simulink library "Vex-V5-Simulink-Expansion"  (R2022a)
settings: Solver=VariableStepAuto  StartTime=0.0  StopTime=10.0  RelTol=1e-3
libraries: $bdroot x48, vexv5lib x31, dspsigops x6, dsparch4 x2, slpidlib x1
(part 1 of 2)
settings Model: Creator=ronan  LastModifiedBy=ronan

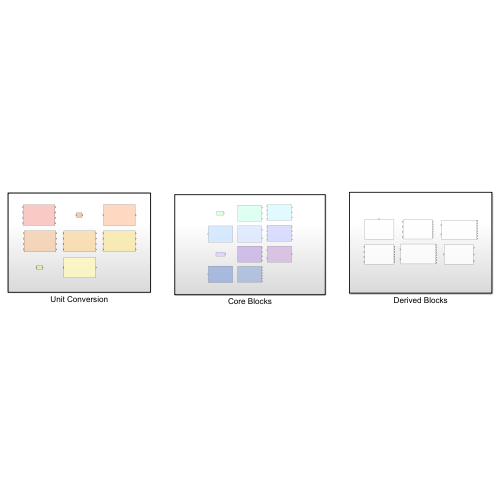
[thumbnail: Simulink's stored preview of the top-level diagram]
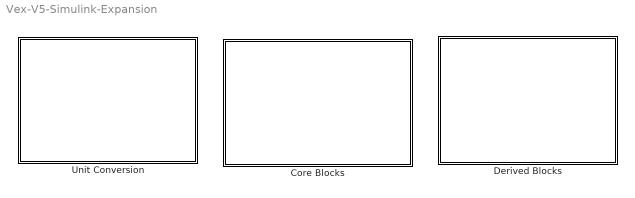
== system Vex-V5-Simulink-Expansion ==
  Core Blocks : Subsystem
  Derived Blocks : Subsystem
  Unit Conversion : Subsystem

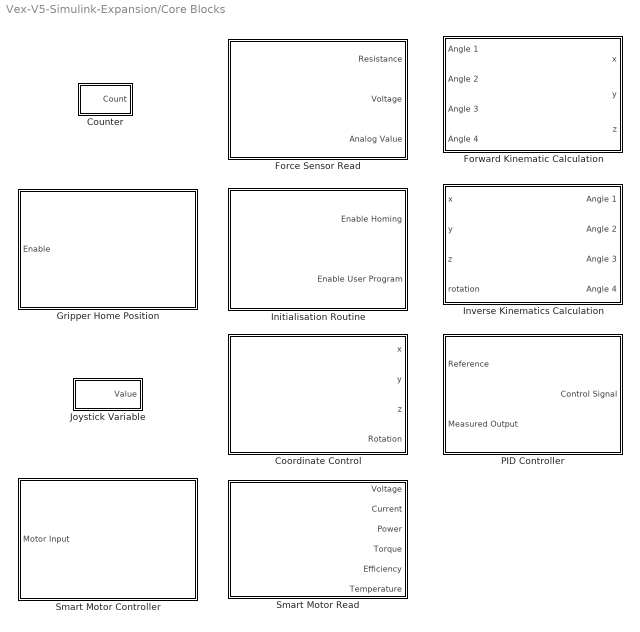
== system Vex-V5-Simulink-Expansion/Core Blocks ==
  Coordinate Control : Subsystem  mask(Coordinate Control){SampleTime=0.01, GX=0, GY=0, GZ=0, GR=0, IX=150, IY=0, IZ=120, IR=85}
      mask prompts: SampleTime "Sample time:"; GX "x (mm/s):"; GY "y (mm/s):"; GZ "z (mm/s):"; GR "Rotation (deg/s):"; IX "x (mm):"; IY "y (mm):"; IZ "z (mm):"; IR "Rotation (deg):"
      mask help: Allows the use of the Vex Joystick's analog sticks as a means to control a Cartesian coordinate and a rotation. This is typically used with the 'Inverse Kinematics Motion' block to allow for manual movement.
      mask TypeOptions SampleTime: Gamepad Joystick/SampleTime | Gamepad Joystick1/SampleTime | Gamepad Joystick2/SampleTime | Gamepad Joystick3/SampleTime
      mask DialogControl ParameterGroupVar Prompt: Global Parameters
      mask DialogControl Container3 Prompt: Maximum Movement Rate
      mask DialogControl Container4 Prompt: Initial Conditions
      mask Display:
      | disp('Coordinate Control');
      | port_label('output', 1, 'x');
      | port_label('output', 2, 'y');
      | port_label('output', 3, 'z');
      | port_label('output', 4, 'Rotation');
  Counter : Subsystem  mask(Counter){SampleTime=0.01, cycleTime=5, cycles=2}
      mask prompts: SampleTime "Sample Time:"; cycleTime "Cycle Time (s):"; cycles "Number of Cycles:"
      mask help: Counts from 1 to the specified limit with the given cycle time before resetting. Outputs the current count.
      mask TypeOptions SampleTime: Delay/SampleTime | Delay1/SampleTime
      mask Display: disp(['Counter']);
  Force Sensor Read : Subsystem  mask(Force Sensor Read){port=H, SampleTime=0.01, Value=22000}
      mask prompts: SampleTime "Sample time:"; Value "Resistance:"
      mask help: Reads the analog input corresponding to the force sensor, and returns the input voltage and the sensor's resistance.
      mask TypeOptions port: Force Sensor Input/port
      mask TypeOptions SampleTime: Force Sensor Input/SampleTime
      mask TypeOptions Value: Resistor Value/Value
      mask DialogControl ParameterGroupVar Prompt: Force Sensor Input
      mask DialogControl Container3 Prompt: Circuit Parameters
      mask Display:
      | port = get_param(gcb, 'port');
      | text(0.4,0.45, ['Input ',port]);
      | text(0.25,0.55, 'Force Sensor Read');
      | port_label('output', 1, 'Resistance');
      | port_label('output', 2, 'Voltage');
      | port_label('output', 3, 'Analog Value');
  Forward Kinematic Calculation : Subsystem  mask(Forward Kinematic Calculation){}
      mask help: Calculates the Cartesian coordinate (mm) of the end effector for a set of motor angles (radians).
      mask Display:
      | disp('Forward Kinematic Calculation');
      | 
      | port_label('output', 1, 'x');
      | port_label('output', 2, 'y');
      | port_label('output', 3, 'z');
      | 
      | port_label('input', 1, 'Angle A');
      | port_label('input', 2, 'Angle B');
      | port_label('input', 3, 'Angle C');
      | port_label('input', 4, 'Angle D');
  Gripper Home Position : Subsystem  mask(Gripper Home Position){SampleTime=0.01, motorPort_right=6, motorPort_left=5}
      mask prompts: SampleTime "Sample Time:"; motorPort_right "Right Gripper:"; motorPort_left "Left Gripper:"
      mask help: Given an enable input, moves the gripper to the home position and resets the motor encoders.
      mask TypeOptions motorPort_right: Subsystem/Right Gripper Read/motorPort | Subsystem/Right Gripper Write/motorPort
      mask TypeOptions motorPort_left: Subsystem/Left Gripper Read/motorPort | Subsystem/Left Gripper Write/motorPort
      mask DialogControl ParameterGroupVar Prompt: Global Parameters
      mask DialogControl Container3 Prompt: Smart Motor Ports
  Initialisation Routine : Subsystem  mask(Initialisation Routine){}
      mask help: Used to home the Vex Arm prior to beginning the User Program - default setting is 5 seconds.
  Inverse Kinematics Calculation : Subsystem  mask(Inverse Kinematics){}
      mask help: Calculates the required motor angles to reach the input end effector rotation (radians) and Cartesian coordinate (mm).
      mask Display:
      | disp('Inverse Kinematic Calculation');
      | 
      | port_label('output', 1, 'Angle A');
      | port_label('output', 2, 'Angle B');
      | port_label('output', 3, 'Angle C');
      | port_label('output', 4, 'Angle D');
      | 
      | port_label('input', 1, 'x');
      | port_label('input', 2, 'y');
      | port_label('input', 3, 'z');
      | port_label('input', 4, 'Rotation');
  Joystick Variable : Subsystem  mask(Joystick Variable){chan_inc=R1, chan_dec=R2, SampleTime=0.01, rate=0, init=0, max=1, min=-1}
      mask prompts: chan_inc "Increment Button:"; chan_dec "Decrement Button:"; SampleTime "Sample time:"; rate "Rate (1/s):"; init "Initial Value:"; max "Maximum Value:"; min "Minimum Value:"
      mask help: Allows a variable to be incremented/decremented using two specified buttons on the Vex Joystick. The rate of change and limits can also be selected.
      mask TypeOptions chan_inc: Gamepad Button Increment/chan
      mask TypeOptions chan_dec: Gamepad Button Decrement/chan
      mask TypeOptions SampleTime: Gamepad Button Decrement/SampleTime | Gamepad Button Increment/SampleTime
      mask DialogControl ParameterGroupVar Prompt: Joystick Parameters
      mask DialogControl Container3 Prompt: Variable Parameters
      mask Display: disp('Variable');
  PID Controller : Subsystem  mask(PID Controller){KP=0, KI=0, KD=0, LimitOutput=off, limitHigh=0, limitLow=0, AntiWindupMode=none, kb=0}
      mask prompts: KP "Proportional (P):"; KI "Integral (I):"; KD "Derivative (D):"; LimitOutput "Simulink:masks:LimitOutput_MP"; limitHigh "Upper limit:"; limitLow "Lower limit:"; AntiWindupMode "Simulink:masks:AntiwindupMethod_MP"; kb "Back-calculation coefficient (Kb):"
      mask help: A general PID controller requiring an input reference and measured value.
      mask TypeOptions LimitOutput: PID/LimitOutput
      mask Callback limitHigh:
      | % Get path to PID controller block
      |     path = strcat(gcb, '/PID');
      |     % Load mask and PID parameters
      |     limMask = get_param(gcb, 'limitHigh');
      |     t = Simulink.Mask.get(path);
      |     limH = t.getParameter('UpperSaturationLimit');
      |     % Set PID limit to mask value
      |     limH.Value = limMask;
      mask Callback limitLow:
      | % Get path to PID controller block
      |     path = strcat(gcb, '/PID');
      |     % Load mask and PID parameters
      |     limMask = get_param(gcb, 'limitLow');
      |     t = Simulink.Mask.get(path);
      |     limL = t.getParameter('LowerSaturationLimit');
      |     % Set PID limit to mask value
      |     limL.Value = limMask;
      mask TypeOptions AntiWindupMode: PID/AntiWindupMode
      mask Callback AntiWindupMode:
      | %{
      |     limMask = get_param(gcb, 'limitOutput');
      |     m = Simulink.Mask.get(gcb);
      |     antiwind = m.getParameter('AntiWindupMode');
      |     kb = m.getParameter('kb');
      |     if strcmp(antiwind.Value,'back-calculation')
      |         if strcmp(limMask,'on')
      |             kb.Enabled = 'on';
      |         end
      |     else
      |         kb.Enabled = 'off';
      |     end
      | %}
      mask Callback kb:
      | % Get path to PID controller block
      |     path = strcat(gcb, '/PID');
      |     % Load mask and PID parameters
      |     kbMask = get_param(gcb, 'kb');
      |     t = Simulink.Mask.get(path);
      |     kbPID = t.getParameter('Kb');
      |     kbPID.Value = kbMask;
      mask DialogControl Container3 Prompt: Controller Parameters
      mask DialogControl ParameterGroupVar Prompt: Output Saturation
      mask DialogControl LimitOutput Prompt: Limit output
      mask DialogControl AntiWindupMode Prompt: Anti-windup Method:
      mask Display:
      | port_label('output', 1, 'Control Signal');
      | port_label('input', 1, 'Reference');
      | port_label('input', 2, 'Measured Output');
      | 
      | kp = get_param(gcb, 'KP');
      | text(0.15,0.1,['KP: ',kp])
      | 
      | ki = get_param(gcb, 'KI');
      | text(0.45,0.1,['KI: ',ki])
      | 
      | kd = get_param(gcb, 'KD');
      | text(0.75,0.1,['KD: ',kd])
  Smart Motor Controller : Subsystem  mask(Smart Motor Controller){motorPort=1, OperationMode=Advanced Control, MotorBrakeMode=Coast}
      mask prompts: motorPort "Smart Port:"; OperationMode "Control Mode:"; MotorBrakeMode "Braking Mode:"
      mask help: Controls the Vex Smart Motor via the chosen method.
      mask TypeOptions motorPort: MATLAB System/motorPort
      mask TypeOptions OperationMode: MATLAB System/OperationMode
      mask TypeOptions MotorBrakeMode: MATLAB System/MotorBrakeMode
      mask DialogControl Container3 Prompt: Smart Motor Configuration
      mask Display:
      | %mode = get_param(gcb, 'control');
      | port = get_param(gcb, 'motorPort');
      | %text(0.3,0.45,[mode]);
      | 
      | text(0.5,0.5, 'Smart Motor Controller','HorizontalAlignment','center');
      | text(0.42,0.15, ['Port: ',port]);
  Smart Motor Read : Subsystem  mask(Smart Motor Read){motorPort=1, SampleTime=0.01}
      mask prompts: motorPort "Smart Port:"; SampleTime "Sample time:"
      mask help: This block reads several attributes relating to the Vex Smart Motors for use in control.
      mask TypeOptions motorPort: MATLAB System1/motorPort
      mask TypeOptions SampleTime: MATLAB System1/SampleTime
      mask Display:
      | port_label('output', 1, 'Voltage');
      | port_label('output', 2, 'Current');
      | port_label('output', 3, 'Power');
      | port_label('output', 4, 'Torque');
      | port_label('output', 5, 'Efficiency');
      | port_label('output', 6, 'Temperature');
      | 
      | text(0.5,0.5,'Smart Motor Read','HorizontalAlignment','center')
      | port = get_param(gcb, 'motorPort');
      | text(0.42,0.15, ['Port: ',port]);

== system Vex-V5-Simulink-Expansion/Derived Blocks ==
  Arm Home Position : Subsystem  mask(Home Position){home_A=0, home_B=0, home_C=0, home_D=0, SampleTime=0.01}
      mask prompts: home_A "Joint A:"; home_B "Joint B:"; home_C "Joint C:"; home_D "Joint D:"; SampleTime "Sample Time:"
      mask help: Moves the Vex Arm into the specified home position prior to executing the user program.
      mask DialogControl ParameterGroupVar Prompt: Potentiometer Home Readings
      mask DialogControl Container3 Prompt: Global Parameters
  Forward Kinematic Motion : Subsystem  mask(Forward Kinematic Motion){SampleTime=0.01, OperationMode=Advanced Control, MotorBrakeMode=Coast, Home_A=0, Home_B=0, Home_C=0, Home_D=0, KP_A=0, KI_A=0, KD_A=0, LimitOutput_A=off, limitHigh_A=0, limitLow_A=0, AntiWindupMode_A=none, kb_A=0, KP_B=0, KI_B=0, KD_B=0, LimitOutput_B=off, limitHigh_B=0, limitLow_B=0, AntiWindupMode_B=none, kb_B=0, KP_C=0, KI_C=0, KD_C=0, LimitOutput_C=off, limitHigh_C=0, limitLow_C=0, AntiWindupMode_C=none, kb_C=0, KP_D=0, KI_D=0, KD_D=0, LimitOutput_D=off, limitHigh_D=0, limitLow_D=0, AntiWindupMode_D=none, kb_D=0}
      mask prompts: SampleTime "Sample Time:"; OperationMode "Control Mode:"; MotorBrakeMode "Braking Mode:"; Home_A "Joint A:"; Home_B "Joint B:"; Home_C "Joint C:"; Home_D "Joint D:"; KP_A "Proportional (P):"; KI_A "Integral (I):"; KD_A "Derivative (D):"; LimitOutput_A "Simulink:masks:LimitOutput_MP"; limitHigh_A "Upper limit:"; limitLow_A "Lower limit:"; AntiWindupMode_A "Simulink:masks:AntiwindupMethod_MP"; kb_A "Back-calculation coefficient (Kb):"; KP_B "Proportional (P):"; KI_B "Integral (I):"; KD_B "Derivative (D):"; LimitOutput_B "Simulink:masks:LimitOutput_MP"; limitHigh_B "Upper limit:"; limitLow_B "Lower limit:"; AntiWindupMode_B "Simulink:masks:AntiwindupMethod_MP"; kb_B "Back-calculation coefficient (Kb):"; KP_C "Proportional (P):"; KI_C "Integral (I):"; KD_C "Derivative (D):"; LimitOutput_C "Simulink:masks:LimitOutput_MP"; limitHigh_C "Upper limit:"; limitLow_C "Lower limit:"; AntiWindupMode_C "Simulink:masks:AntiwindupMethod_MP"; kb_C "Back-calculation coefficient (Kb):"; KP_D "Proportional (P):"; KI_D "Integral (I):"; KD_D "Derivative (D):"; LimitOutput_D "Simulink:masks:LimitOutput_MP"; limitHigh_D "Upper limit:"; limitLow_D "Lower limit:"; AntiWindupMode_D "Simulink:masks:AntiwindupMethod_MP"; kb_D "Back-calculation coefficient (Kb):"
      mask help: Given a set of 4 arm angles (radians), moves the arm into that position using the selected PID control parameters and outputs the current pose and Cartesian coordinate of the end effector (mm).
      mask TypeOptions OperationMode: Smart Motor Controller A/OperationMode | Smart Motor Controller B/OperationMode | Smart Motor Controller C/OperationMode | Smart Motor Controller D/OperationMode
      mask TypeOptions MotorBrakeMode: Smart Motor Controller A/MotorBrakeMode | Smart Motor Controller B/MotorBrakeMode | Smart Motor Controller C/MotorBrakeMode | Smart Motor Controller D/MotorBrakeMode
      mask TypeOptions Home_A: A2P/Home_A | P2A/Home_A
      mask TypeOptions Home_B: A2P/Home_B | P2A/Home_B
      mask TypeOptions Home_C: A2P/Home_C | P2A/Home_C
      mask TypeOptions Home_D: A2P/Home_D | P2A/Home_D
      mask TypeOptions KP_A: PID Controller A/KP
      mask TypeOptions KI_A: PID Controller A/KI
      mask TypeOptions KD_A: PID Controller A/KD
      mask TypeOptions LimitOutput_A: PID Controller A/LimitOutput
      mask TypeOptions limitHigh_A: PID Controller A/limitHigh
      mask TypeOptions limitLow_A: PID Controller A/limitLow
      mask TypeOptions AntiWindupMode_A: PID Controller A/AntiWindupMode
      mask TypeOptions kb_A: PID Controller A/kb
      mask TypeOptions KP_B: PID Controller B/KP
      mask TypeOptions KI_B: PID Controller B/KI
      mask TypeOptions KD_B: PID Controller B/KD
      mask TypeOptions LimitOutput_B: PID Controller B/LimitOutput
      mask TypeOptions limitHigh_B: PID Controller B/limitHigh
      mask TypeOptions limitLow_B: PID Controller B/limitLow
      mask TypeOptions AntiWindupMode_B: PID Controller B/AntiWindupMode
      mask TypeOptions kb_B: PID Controller B/kb
      mask TypeOptions KP_C: PID Controller C/KP
      mask TypeOptions KI_C: PID Controller C/KI
      mask TypeOptions KD_C: PID Controller C/KD
      mask TypeOptions LimitOutput_C: PID Controller C/LimitOutput
      mask TypeOptions limitHigh_C: PID Controller C/limitHigh
      mask TypeOptions limitLow_C: PID Controller C/limitLow
      mask TypeOptions AntiWindupMode_C: PID Controller C/AntiWindupMode
      mask TypeOptions kb_C: PID Controller C/kb
      mask TypeOptions KP_D: PID Controller D/KP
      mask TypeOptions KI_D: PID Controller D/KI
      mask TypeOptions KD_D: PID Controller D/KD
      mask TypeOptions LimitOutput_D: PID Controller D/LimitOutput
      mask TypeOptions limitHigh_D: PID Controller D/limitHigh
      mask TypeOptions limitLow_D: PID Controller D/limitLow
      mask TypeOptions AntiWindupMode_D: PID Controller D/AntiWindupMode
      mask TypeOptions kb_D: PID Controller D/kb
      mask DialogControl Container17 Prompt: Global Parameters
      mask DialogControl Container16 Prompt: Global Motor Parameters
      mask DialogControl Container15 Prompt: Potentiometer Home Values
      mask DialogControl Container3 Prompt: PID Controller A
      mask DialogControl Container7 Prompt: PID Gains
      mask DialogControl Container8 Prompt: Output Saturation
      mask DialogControl LimitOutput_A Prompt: Limit output
      mask DialogControl AntiWindupMode_A Prompt: Anti-windup Method:
      mask DialogControl Container4 Prompt: PID Controller B
      mask DialogControl Container9 Prompt: PID Gains
      mask DialogControl Container10 Prompt: Output Saturation
      mask DialogControl LimitOutput_B Prompt: Limit output
      mask DialogControl AntiWindupMode_B Prompt: Anti-windup Method:
      mask DialogControl Container5 Prompt: PID Controller C
      mask DialogControl Container11 Prompt: PID Gains
      mask DialogControl Container12 Prompt: Output Saturation
      mask DialogControl LimitOutput_C Prompt: Limit output
      mask DialogControl AntiWindupMode_C Prompt: Anti-windup Method:
      mask DialogControl Container6 Prompt: PID Controller D
      mask DialogControl Container13 Prompt: PID Gains
      mask DialogControl Container14 Prompt: Output Saturation
      mask DialogControl LimitOutput_D Prompt: Limit output
      mask DialogControl AntiWindupMode_D Prompt: Anti-windup Method:
  Individual Gripper Control : Subsystem  mask(Individual Gripper Control){SampleTime=0.01, motorPort_right=5, motorPort_left=6, KP=0, KI=0, KD=0, LimitOutput=off, limitHigh=0, limitLow=0, AntiWindupMode=none, kb=0, fsr_unit=Resistance, port_LA=A, LA=47000, port_LB=B, LB=47000, port_RA=D, RA=47000, port_RB=C, RB=47000}
      mask prompts: SampleTime "Sample Time:"; motorPort_right "Right Smart Port:"; motorPort_left "Left Smart Port:"; KP "Proportional (P):"; KI "Integral (I):"; KD "Derivative (D):"; LimitOutput "Simulink:masks:LimitOutput_MP"; limitHigh "Upper limit:"; limitLow "Lower limit:"; AntiWindupMode "Simulink:masks:AntiwindupMethod_MP"; kb "Back-calculation coefficient (Kb):"; fsr_unit "Output Unit:"; port_LA "Port:"; LA "Resistance:"; port_LB "Port:"; LB "Resistance:"; port_RA "Port:"; RA "Resistance:"; port_RB "Port:"; RB "Resistance:"
      mask help: Allows control of each gripper arm's position via a reference angle and PID parameters. Returns force sensor readings, the current motor encoder positions and the measured torque.
      mask TypeOptions motorPort_right: Right Smart Motor Controller/motorPort | Smart Motor Read Right/motorPort
      mask TypeOptions motorPort_left: Left Smart Motor Controller/motorPort | Smart Motor Read Left/motorPort
      mask TypeOptions KP: PID Controller Left/KP | PID Controller Right/KP
      mask TypeOptions KI: PID Controller Left/KI | PID Controller Right/KI
      mask TypeOptions KD: PID Controller Left/KD | PID Controller Right/KD
      mask TypeOptions LimitOutput: PID Controller Left/LimitOutput | PID Controller Right/LimitOutput
      mask TypeOptions limitHigh: PID Controller Left/limitHigh | PID Controller Right/limitHigh
      mask TypeOptions limitLow: PID Controller Left/limitLow | PID Controller Right/limitLow
      mask TypeOptions AntiWindupMode: PID Controller Left/AntiWindupMode | PID Controller Right/AntiWindupMode
      mask TypeOptions kb: PID Controller Left/kb | PID Controller Right/kb
      mask TypeOptions fsr_unit: Resistance | Voltage | Analog Reading
      mask TypeOptions port_LA: FSR Left 1/port
      mask TypeOptions LA: FSR Left 1/Value
      mask TypeOptions port_LB: FSR Left 2/port
      mask TypeOptions LB: FSR Left 2/Value
      mask TypeOptions port_RA: FSR Right 1/port
      mask TypeOptions RA: FSR Right 1/Value
      mask TypeOptions port_RB: FSR Right 2/port
      mask TypeOptions RB: FSR Right 2/Value
      mask DialogControl ParameterGroupVar Prompt: Global Parameters
      mask DialogControl Container15 Prompt: Motor Parameters
      mask DialogControl Container7 Prompt: Position PID Controller
      mask DialogControl Container4 Prompt: PID Gains
      mask DialogControl Container5 Prompt: Output Saturation
      mask DialogControl LimitOutput Prompt: Limit output
      mask DialogControl AntiWindupMode Prompt: Anti-windup Method:
      mask DialogControl Container8 Prompt: Force Sensor Reading
      mask DialogControl Container11 Prompt: Left A
      mask DialogControl Container12 Prompt: Left B
      mask DialogControl Container9 Prompt: Right A
      mask DialogControl Container10 Prompt: Right B
  Inverse Kinematic Motion : Subsystem  mask(Inverse Kinematic Motion){SampleTime=0.01, MotorBrakeMode=Coast, OperationMode=Advanced Control, Home_A=0, Home_B=0, Home_C=0, Home_D=0, KP_A=0, KI_A=0, KD_A=0, limitOutput_A=off, limitHigh_A=0, limitLow_A=0, AntiWindupMode_A=none, kb_A=0, KP_B=0, KI_B=0, KD_B=0, limitOutput_B=off, limitHigh_B=0, limitLow_B=0, AntiWindupMode_B=none, kb_B=0, KP_C=0, KI_C=0, KD_C=0, limitOutput_C=off, limitHigh_C=0, limitLow_C=0, AntiWindupMode_C=none, kb_C=0, KP_D=0, KI_D=0, KD_D=0, limitOutput_D=off, limitHigh_D=0, limitLow_D=0, AntiWindupMode_D=none, kb_D=0}
      mask prompts: SampleTime "Sample Time:"; MotorBrakeMode "Braking Mode:"; OperationMode "Control Mode:"; Home_A "Joint A:"; Home_B "Joint B:"; Home_C "Joint C:"; Home_D "Joint D:"; KP_A "Proportional (P):"; KI_A "Integral (I):"; KD_A "Derivative (D):"; limitOutput_A "Limit output:"; limitHigh_A "Upper limit:"; limitLow_A "Lower limit:"; AntiWindupMode_A "Simulink:masks:AntiwindupMethod_MP"; kb_A "Back-calculation coefficient (Kb):"; KP_B "Proportional (P):"; KI_B "Integral (I):"; KD_B "Derivative (D):"; limitOutput_B "Limit output:"; limitHigh_B "Upper limit:"; limitLow_B "Lower limit:"; AntiWindupMode_B "Simulink:masks:AntiwindupMethod_MP"; kb_B "Back-calculation coefficient (Kb):"; KP_C "Proportional (P):"; KI_C "Integral (I):"; KD_C "Derivative (D):"; limitOutput_C "Limit output:"; limitHigh_C "Upper limit:"; limitLow_C "Lower limit:"; AntiWindupMode_C "Simulink:masks:AntiwindupMethod_MP"; kb_C "Back-calculation coefficient (Kb):"; KP_D "Proportional (P):"; KI_D "Integral (I):"; KD_D "Derivative (D):"; limitOutput_D "Limit output:"; limitHigh_D "Upper limit:"; limitLow_D "Lower limit:"; AntiWindupMode_D "Simulink:masks:AntiwindupMethod_MP"; kb_D "Back-calculation coefficient (Kb):"
      mask help: Given a cartesian coordinate and rotation for the end effector, calculates the required motor angles and moves the arm into that position using the selected PID control parameters.
      mask TypeOptions MotorBrakeMode: Smart Motor Controller A/MotorBrakeMode | Smart Motor Controller B/MotorBrakeMode | Smart Motor Controller C/MotorBrakeMode | Smart Motor Controller D/MotorBrakeMode
      mask TypeOptions OperationMode: Smart Motor Controller A/OperationMode | Smart Motor Controller B/OperationMode | Smart Motor Controller C/OperationMode | Smart Motor Controller D/OperationMode
      mask TypeOptions Home_A: A2P/Home_A | P2A/Home_A
      mask TypeOptions Home_B: A2P/Home_B | P2A/Home_B
      mask TypeOptions Home_C: A2P/Home_C | P2A/Home_C
      mask TypeOptions Home_D: A2P/Home_D | P2A/Home_D
      mask TypeOptions KP_A: PID Controller A/KP
      mask TypeOptions KI_A: PID Controller A/KI
      mask TypeOptions KD_A: PID Controller A/KD
      mask TypeOptions limitOutput_A: PID Controller A/limitOutput
      mask TypeOptions limitHigh_A: PID Controller A/limitHigh
      mask TypeOptions limitLow_A: PID Controller A/limitLow
      mask TypeOptions AntiWindupMode_A: PID Controller A/AntiWindupMode
      mask TypeOptions kb_A: PID Controller A/kb
      mask TypeOptions KP_B: PID Controller B/KP
      mask TypeOptions KI_B: PID Controller B/KI
      mask TypeOptions KD_B: PID Controller B/KD
      mask TypeOptions limitOutput_B: PID Controller B/limitOutput
      mask TypeOptions limitHigh_B: PID Controller B/limitHigh
      mask TypeOptions limitLow_B: PID Controller B/limitLow
      mask TypeOptions AntiWindupMode_B: PID Controller B/AntiWindupMode
      mask TypeOptions kb_B: PID Controller B/kb
      mask TypeOptions KP_C: PID Controller C/KP
      mask TypeOptions KI_C: PID Controller C/KI
      mask TypeOptions KD_C: PID Controller C/KD
      mask TypeOptions limitOutput_C: PID Controller C/limitOutput
      mask TypeOptions limitHigh_C: PID Controller C/limitHigh
      mask TypeOptions limitLow_C: PID Controller C/limitLow
      mask TypeOptions AntiWindupMode_C: PID Controller C/AntiWindupMode
      mask TypeOptions kb_C: PID Controller C/kb
      mask TypeOptions KP_D: PID Controller D/KP
      mask TypeOptions KI_D: PID Controller D/KI
      mask TypeOptions KD_D: PID Controller D/KD
      mask TypeOptions limitOutput_D: PID Controller D/limitOutput
      mask TypeOptions limitHigh_D: PID Controller D/limitHigh
      mask TypeOptions limitLow_D: PID Controller D/limitLow
      mask TypeOptions AntiWindupMode_D: PID Controller D/AntiWindupMode
      mask TypeOptions kb_D: PID Controller D/kb
      mask DialogControl Container17 Prompt: Global Parameters
      mask DialogControl ParameterGroupVar Prompt: Global Motor Parameters
      mask DialogControl Container16 Prompt: Potentiometer Home Values
      mask DialogControl Container4 Prompt: PID Controller A
      mask DialogControl Container8 Prompt: PID Gains
      mask DialogControl Container9 Prompt: Output Saturation
      mask DialogControl AntiWindupMode_A Prompt: Anti-windup Method:
      mask DialogControl Container5 Prompt: PID Controller B
      mask DialogControl Container10 Prompt: PID Gains
      mask DialogControl Container11 Prompt: Output Saturation
      mask DialogControl AntiWindupMode_B Prompt: Anti-windup Method:
      mask DialogControl Container6 Prompt: PID Controller C
      mask DialogControl Container12 Prompt: PID Gains
      mask DialogControl Container13 Prompt: Output Saturation
      mask DialogControl AntiWindupMode_C Prompt: Anti-windup Method:
      mask DialogControl Container7 Prompt: PID Controller D
      mask DialogControl Container14 Prompt: PID Gains
      mask DialogControl Container15 Prompt: Output Saturation
      mask DialogControl AntiWindupMode_D Prompt: Anti-windup Method:
  Joint Gripper Control : Subsystem  mask(Joint Gripper Control){SampleTime=0.01, motorPort_right=6, motorPort_left=5, KP_position=0, KI_positon=0, KD_position=0, LimitOutput_position=off, limitHigh_position=0, limitLow_position=0, AntiWindupMode_position=none, kb_position=0, KP=0, KI=0, KD=0, LimitOutput=off, limitHigh=0, limitLow=0, AntiWindupMode=none, kb=0, LA=10000, port_LA=H, LB=10000, port_LB=G, RA=10000, port_RA=F, RB=10000, port_RB=E, fsr_unit=Resistance}
      mask prompts: SampleTime "Sample Time:"; motorPort_right "Right Smart Port:"; motorPort_left "Left Smart Port:"; KP_position "Proportional (P):"; KI_positon "Integral (I):"; KD_position "Derivative (D):"; LimitOutput_position "Simulink:masks:LimitOutput_MP"; limitHigh_position "Upper limit:"; limitLow_position "Lower limit:"; AntiWindupMode_position "Simulink:masks:AntiwindupMethod_MP"; kb_position "Back-calculation coefficient (Kb):"; KP "Proportional (P):"; KI "Integral (I):"; KD "Derivative (D):"; LimitOutput "Simulink:masks:LimitOutput_MP"; limitHigh "Upper limit:"; limitLow "Lower limit:"; AntiWindupMode "Simulink:masks:AntiwindupMethod_MP"; kb "Back-calculation coefficient (Kb):"; LA "Resistance:"; port_LA "Port:"; LB "Resistance:"; port_LB "Port:"; RA "Resistance:"; port_RA "Port:"; RB "Resistance:"; port_RB "Port:"; fsr_unit "Output Unit:"
      mask help: Allows joint control of the gripper position via a reference angle and PID parameters, and joint control of the gripper torque via a reference torque and another set of PID parameters. Returns force sensor readings, the current motor encoder positions and the measured torque.
      mask TypeOptions motorPort_right: Right Torque/motorPort | Smart Motor Controller Right/motorPort | Smart Motor Read Right/motorPort
      mask TypeOptions motorPort_left: Left Torque/motorPort | Smart Motor Controller Left/motorPort | Smart Motor Read Left/motorPort
      mask TypeOptions KP_position: PID Controller Position/KP
      mask TypeOptions KI_positon: PID Controller Position/KI
      mask TypeOptions KD_position: PID Controller Position/KD
      mask TypeOptions LimitOutput_position: PID Controller Position/LimitOutput
      mask TypeOptions limitHigh_position: PID Controller Position/limitHigh
      mask TypeOptions limitLow_position: PID Controller Position/limitLow
      mask TypeOptions AntiWindupMode_position: PID Controller Position/AntiWindupMode
      mask TypeOptions kb_position: PID Controller Position/kb
      mask TypeOptions KP: PID Controller Torque/KP
      mask TypeOptions KI: PID Controller Torque/KI
      mask TypeOptions KD: PID Controller Torque/KD
      mask TypeOptions LimitOutput: PID Controller Torque/LimitOutput
      mask TypeOptions limitHigh: PID Controller Torque/limitHigh
      mask TypeOptions limitLow: PID Controller Torque/limitLow
      mask TypeOptions AntiWindupMode: PID Controller Torque/AntiWindupMode
      mask TypeOptions kb: PID Controller Torque/kb
      mask TypeOptions LA: FSR Left 1/Value
      mask TypeOptions port_LA: FSR Left 1/port
      mask TypeOptions LB: FSR Left 2/Value
      mask TypeOptions port_LB: FSR Left 2/port
      mask TypeOptions RA: FSR Right 1/Value
      mask TypeOptions port_RA: FSR Right 1/port
      mask TypeOptions RB: FSR Right 2/Value
      mask TypeOptions port_RB: FSR Right 2/port
      mask TypeOptions fsr_unit: Resistance | Voltage | Analog Reading
      mask DialogControl Container18 Prompt: Global Parameters
      mask DialogControl Container19 Prompt: Motor Parameters
      mask DialogControl Container4 Prompt: Position PID Controller
      mask DialogControl Container17 Prompt: PID Gains
      mask DialogControl Container8 Prompt: Output Saturation
      mask DialogControl LimitOutput_position Prompt: Limit output
      mask DialogControl AntiWindupMode_position Prompt: Anti-windup Method:
      mask DialogControl Container3 Prompt: Torque PID Controller
      mask DialogControl Container7 Prompt: PID Gains
      mask DialogControl Container9 Prompt: Output Saturation
      mask DialogControl LimitOutput Prompt: Limit output
      mask DialogControl AntiWindupMode Prompt: Anti-windup Method:
      mask DialogControl Container12 Prompt: Force Sensor Reading
      mask DialogControl Container16 Prompt: FSR Left A
      mask DialogControl Container15 Prompt: FSR Left B
      mask DialogControl Container14 Prompt: FSR Right A
      mask DialogControl Container13 Prompt: FSR Right B
  Motor Torque Control : Subsystem  mask(Motor Torque Control){motorPort=5, SampleTime=0.01, KP=0, KI=0, KD=0, limitOutput=off, limitHigh=0, limitLow=0, AntiWindupMode=none, kb=0}
      mask prompts: motorPort "Smart Port:"; SampleTime "Sample time:"; KP "Proportional (P):"; KI "Integral (I):"; KD "Derivative (D):"; limitOutput "Limit output:"; limitHigh "Upper limit:"; limitLow "Lower limit:"; AntiWindupMode "Simulink:masks:AntiwindupMethod_MP"; kb "Back-calculation coefficient (Kb):"
      mask help: Uses a PID controller to match the reference torque of the specified Smart Motor. The PID contoller outputs a voltage to control the Smart Motor.
      mask TypeOptions motorPort: Motor Read/motorPort | Smart Motor Controller/motorPort
      mask TypeOptions SampleTime: Motor Read/SampleTime
      mask TypeOptions KP: PID/KP
      mask TypeOptions KI: PID/KI
      mask TypeOptions KD: PID/KD
      mask TypeOptions limitOutput: PID/limitOutput
      mask TypeOptions limitHigh: PID/limitHigh
      mask TypeOptions limitLow: PID/limitLow
      mask TypeOptions AntiWindupMode: PID/AntiWindupMode
      mask TypeOptions kb: PID/kb
      mask DialogControl ParameterGroupVar Prompt: Smart Motor Parameters
      mask DialogControl Container3 Prompt: PID Controller
      mask DialogControl Container4 Prompt: PID Gains
      mask DialogControl Container5 Prompt: Output Saturation
      mask DialogControl AntiWindupMode Prompt: Anti-windup Method:

== system Vex-V5-Simulink-Expansion/Unit Conversion ==
  Angle to Potentiometer Reading : Subsystem  mask(Angle to Potentiometer Reading){Home_A=0, Home_B=0, Home_C=0, Home_D=0}
      mask prompts: Home_A "Joint A:"; Home_B "Joint B:"; Home_C "Joint C:"; Home_D "Joint D:"
      mask help:
      | Converts a set of Vex Arm member angles into potentiometer readings. Requires the potentiometer readings taken with the home
      |  jig insterted.
      mask TypeOptions Home_A: Home A/Value
      mask TypeOptions Home_B: Home B/Value
      mask TypeOptions Home_C: Home C/Value
      mask TypeOptions Home_D: Home D/Value
      mask DialogControl ParameterGroupVar Prompt: Potentiometer Home Readings
      mask Display:
      | disp('A2P');
      | 
      | 
      | port_label('output', 1, 'Target A');
      | port_label('output', 2, 'Target B');
      | port_label('output', 3, 'Target C');
      | port_label('output', 4, 'Target D');
      | 
      | port_label('input', 1, 'Angle A');
      | port_label('input', 2, 'Angle B');
      | port_label('input', 3, 'Angle C');
      | port_label('input', 4, 'Angle D');
  Force to Resistance : Subsystem  mask(Force to Resistance){m=0, K=0}
      mask prompts: m "Gradient (m):"; K "Constant (K):"
      mask help: Converts a force (N) into an equivalent force sensor resistance (Ohms) using the gradient and intercept of the linear log-log plot.
  Joint to Motor Angle : Subsystem  mask(Joint to Motor Angle){}
      mask help: Converts Vex Arm joint angles to motor angles (radians).
  Motor to Joint Angle : Subsystem  mask(Motor to Joint Angle){}
      mask help: Converts Vex Arm motor angles to joint angles (radians).
  Potentiometer Reading to Angle : Subsystem  mask(Potentiometer Reading to Analog){Home_A=0, Home_B=0, Home_C=0, Home_D=0}
      mask prompts: Home_A "Joint A:"; Home_B "Joint B:"; Home_C "Joint C:"; Home_D "Joint D:"
      mask help:
      | Converts a set of potentiometer readings into Vex Arm member angles. Requires the potentiometer readings taken with the home
      |  jig insterted.
      mask DialogControl ParameterGroupVar Prompt: Potentiometer Home Readings
      mask Display:
      | disp('P2A');
      | 
      | port_label('output', 1, 'Angle A');
      | port_label('output', 2, 'Angle B');
      | port_label('output', 3, 'Angle C');
      | port_label('output', 4, 'Angle D');
      | 
      | port_label('input', 1, 'Reading A');
      | port_label('input', 2, 'Reading B');
      | port_label('input', 3, 'Reading C');
      | port_label('input', 4, 'Reading D');
  Resistance to Force : Subsystem  mask(Resistance to Force){m=0, K=0}
      mask prompts: m "Gradient (m):"; K "Constant (K):"
      mask help: Converts the resistance (Ohms) of a force sensor into a force (N) using the gradient and intercept of the linear log-log plot.
  deg2Rad : Subsystem  mask(Degrees to Radians){}
      mask help: Converts an input angle in degrees to radians.
      mask Display: disp('D2R');
  rad2Deg : Subsystem  mask(Radians to Degrees){}
      mask help: Converts an input angle in radians to degrees.
      mask Display: disp('R2D');

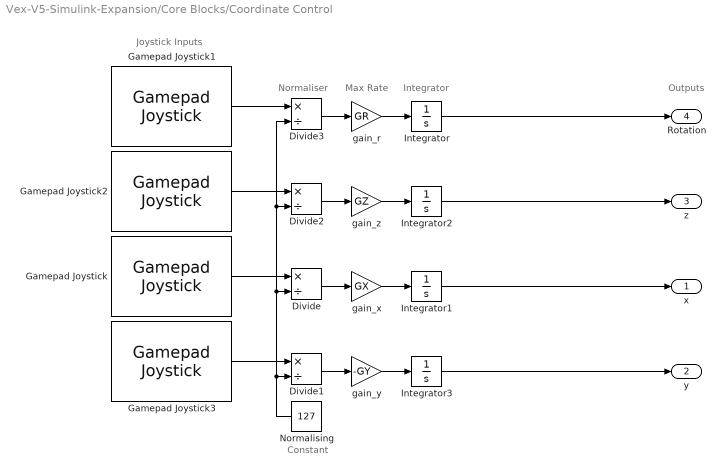
== system Vex-V5-Simulink-Expansion/Core Blocks/Coordinate Control ==
  note: Normaliser
  note: Integrator
  note: Max Rate
  note: Outputs
  note: Constant
  note: Joystick Inputs
  Divide{,1..3} (4 alike) : Product  Inputs=*/
  Gamepad Joystick : vexv5lib/Gamepad/Gamepad Joystick  joystickType=Primary  chan=3  SampleTime=SampleTime
      settings: SourceProductBaseCode=VEXV5
  Gamepad Joystick1 : vexv5lib/Gamepad/Gamepad Joystick  joystickType=Primary  chan=1  SampleTime=SampleTime
      settings: SourceProductBaseCode=VEXV5
  Gamepad Joystick2 : vexv5lib/Gamepad/Gamepad Joystick  joystickType=Primary  chan=2  SampleTime=SampleTime
      settings: SourceProductBaseCode=VEXV5
  Gamepad Joystick3 : vexv5lib/Gamepad/Gamepad Joystick  joystickType=Primary  chan=4  SampleTime=SampleTime
      settings: SourceProductBaseCode=VEXV5
  Integrator : Integrator  InitialCondition=IR
  Integrator1 : Integrator  InitialCondition=IX  LimitOutput=on  UpperSaturationLimit=300  LowerSaturationLimit=0
  Integrator2 : Integrator  InitialCondition=IZ  LimitOutput=on  LowerSaturationLimit=100
  Integrator3 : Integrator  InitialCondition=IY  LowerSaturationLimit=0
  Normalising : Constant  Value=127
  gain_r : Gain  Gain=GR
  gain_x : Gain  Gain=GX
  gain_y : Gain  Gain=-GY
  gain_z : Gain  Gain=GZ
  x : Outport
  y : Outport  Port=2
  z : Outport  Port=3
  Rotation : Outport  Port=4
  wires:
  Normalising/1 -> Divide1/2, Divide/2, Divide2/2, Divide3/2
  gain_r/1 -> Integrator/1
  Divide3/1 -> gain_r/1
  Gamepad Joystick1/1 -> Divide3/1
  Gamepad Joystick2/1 -> Divide2/1
  Divide2/1 -> gain_z/1
  gain_z/1 -> Integrator2/1
  Gamepad Joystick3/1 -> Divide1/1
  Divide1/1 -> gain_y/1
  gain_y/1 -> Integrator3/1
  gain_x/1 -> Integrator1/1
  Divide/1 -> gain_x/1
  Gamepad Joystick/1 -> Divide/1
  Integrator1/1 -> x/1
  Integrator2/1 -> z/1
  Integrator/1 -> Rotation/1
  Integrator3/1 -> y/1

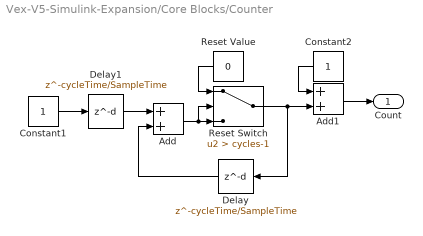
== system Vex-V5-Simulink-Expansion/Core Blocks/Counter ==
  Add : Sum
  Add1 : Sum
  Constant1 : Constant
  Constant2 : Constant
  Delay : Delay  DelayLength=cycleTime/SampleTime  SampleTime=SampleTime
  Delay1 : Delay  DelayLength=cycleTime/SampleTime  SampleTime=SampleTime
  Reset Switch : Switch  Criteria=u2 > Threshold  Threshold=cycles-1  SaturateOnIntegerOverflow=off  InputSameDT=off
  Reset Value : Constant  Value=0
  Count : Outport
  wires:
  Reset Value/1 -> Reset Switch/1
  Add/1 -> Reset Switch/2, Reset Switch/3
  Reset Switch/1 -> Add1/2, Delay/1
  Delay/1 -> Add/2
  Delay1/1 -> Add/1
  Constant1/1 -> Delay1/1
  Add1/1 -> Count/1
  Constant2/1 -> Add1/1

== system Vex-V5-Simulink-Expansion/Core Blocks/Force Sensor Read ==
  note: Outputs
  Divide : Product  Inputs=**/
  Force Sensor Input : vexv5lib/Sensors/Analog Input  port=H  SampleTime=SampleTime
      settings: SourceProductBaseCode=VEXV5
  MATLAB Function : MATLAB Function  TreatAsAtomicUnit=on
  Max Voltage : Constant  Value=5
  Resistor Value : Constant  Value=Value
  Resolution : Constant  Value=4095
  Resistance : Outport
  Voltage : Outport  Port=2
  Analog Value : Outport  Port=3
  wires:
  Divide/1 -> Voltage/1, MATLAB Function/2(volOut)
  Resolution/1 -> Divide/3
  Resistor Value/1 -> MATLAB Function/3(res)
  Force Sensor Input/1 -> Analog Value/1, Divide/2
  MATLAB Function/1(forceRes) -> Resistance/1
  Max Voltage/1 -> MATLAB Function/1(volIn), Divide/1

== system Vex-V5-Simulink-Expansion/Core Blocks/Forward Kinematic Calculation ==
  note: Outputs
  note: Inputs
  Angle 1 : Inport
  Angle 2 : Inport  Port=2
  Angle 3 : Inport  Port=3
  Angle 4 : Inport  Port=4
  MATLAB Function5 : MATLAB Function  TreatAsAtomicUnit=on
  x : Outport
  y : Outport  Port=2
  z : Outport  Port=3
  wires:
  Angle 1/1 -> MATLAB Function5/1(a1)
  Angle 2/1 -> MATLAB Function5/2(a2)
  Angle 3/1 -> MATLAB Function5/3(a3)
  Angle 4/1 -> MATLAB Function5/4(a4)
  MATLAB Function5/1(x) -> x/1
  MATLAB Function5/2(y) -> y/1
  MATLAB Function5/3(z) -> z/1

== system Vex-V5-Simulink-Expansion/Core Blocks/Gripper Home Position ==
  Enable : Inport
  Subsystem : Subsystem
  wires:
  Enable/1 -> Subsystem/Enable

== system Vex-V5-Simulink-Expansion/Core Blocks/Initialisation Routine ==
  Clock : Clock
  Initialisation Schedule : Stateflow chart  TreatAsAtomicUnit=on
  Enable Homing : Outport
  Enable User Program : Outport  Port=2
  wires:
  Clock/1 -> Initialisation Schedule/1(simulation_time)
  Initialisation Schedule/1(enable_homing) -> Enable Homing/1
  Initialisation Schedule/2(enable_user) -> Enable User Program/1

== system Vex-V5-Simulink-Expansion/Core Blocks/Inverse Kinematics Calculation ==
  note: Outputs
  note: Inputs
  x : Inport
  y : Inport  Port=2
  z : Inport  Port=3
  rotation : Inport  Port=4
  MATLAB Function : MATLAB Function  TreatAsAtomicUnit=on
  Angle 1 : Outport
  Angle 2 : Outport  Port=2
  Angle 3 : Outport  Port=3
  Angle 4 : Outport  Port=4
  wires:
  MATLAB Function/1(a1) -> Angle 1/1
  MATLAB Function/2(a2) -> Angle 2/1
  MATLAB Function/3(a3) -> Angle 3/1
  MATLAB Function/4(a4) -> Angle 4/1
  x/1 -> MATLAB Function/1(x)
  y/1 -> MATLAB Function/2(y)
  z/1 -> MATLAB Function/3(z)
  rotation/1 -> MATLAB Function/4(rotation)

== system Vex-V5-Simulink-Expansion/Core Blocks/Joystick Variable ==
  note: Integrator
  note: Max Rate
  note: Output
  Add : Sum  Inputs=+-
  Gamepad Button Decrement : vexv5lib/Gamepad/Gamepad Button  joystickType=Primary  chan=R2  SampleTime=SampleTime
      settings: SourceProductBaseCode=VEXV5
  Gamepad Button Increment : vexv5lib/Gamepad/Gamepad Button  joystickType=Primary  chan=R1  SampleTime=SampleTime
      settings: SourceProductBaseCode=VEXV5
  Integrator : Integrator  InitialCondition=init  LimitOutput=on  UpperSaturationLimit=max  LowerSaturationLimit=min
  gain_r : Gain  Gain=rate
  Value : Outport
  wires:
  gain_r/1 -> Integrator/1
  Gamepad Button Increment/1 -> Add/1
  Gamepad Button Decrement/1 -> Add/2
  Add/1 -> gain_r/1
  Integrator/1 -> Value/1

== system Vex-V5-Simulink-Expansion/Core Blocks/PID Controller ==
  note: Output
  note: Inputs
  Reference : Inport
  Measured Output : Inport  Port=2
  PID : slpidlib/PID Controller  Controller=PID  Form=Parallel  TimeDomain=Discrete-time  UseExternalTs=off  SampleTime=-1  IntegratorMethod=Forward Euler  FilterMethod=Forward Euler  ControllerParametersSource=internal  P=KP  I=KI  UseKiTs=off  D=KD  N=100  UseFilter=on  TunerSelectOption=Transfer Function Based (PID Tuner App)  InitialConditionSource=internal  InitialConditionForIntegrator=0  InitialConditionForFilter=0  DifferentiatorICPrevScaledInput=0  ExternalReset=none  TrackingMode=off  Kt=1  LimitOutput=off  SatLimitsSource=internal  UpperSaturationLimit=0  LowerSaturationLimit=0  LinearizeAsGain=on  AntiWindupMode=none  Kb=0  POutMin=[]  POutMax=[]  IOutMin=[]  IOutMax=[]  DOutMin=[]  DOutMax=[]  NOutMin=[]  NOutMax=[]  SumOutMin=[]  SumOutMax=[]  SaturationOutMin=[]  SaturationOutMax=[]  PParamMin=[]  PParamMax=[]  IParamMin=[]  IParamMax=[]  DParamMin=[]  DParamMax=[]  NParamMin=[]  NParamMax=[]  KbParamMin=[]  KbParamMax=[]  KtParamMin=[]  KtParamMax=[]  KbOutMin=[]  KbOutMax=[]  KtOutMin=[]  KtOutMax=[]  IntegratorOutMin=[]  IntegratorOutMax=[]  FilterOutMin=[]  FilterOutMax=[]  SumI1OutMin=[]  SumI1OutMax=[]  SumI2OutMin=[]  SumI2OutMax=[]  SumI3OutMin=[]  SumI3OutMax=[]  SumI4OutMin=[]  SumI4OutMax=[]  SumDOutMin=[]  SumDOutMax=[]  DifferentiatorOutMin=[]  DifferentiatorOutMax=[]  FilterDiffOutCoefMin=[]  FilterDiffOutCoefMax=[]  ReciprocalOutMin=[]  ReciprocalOutMax=[]  SumDenOutMin=[]  SumDenOutMax=[]  SumNumOutMin=[]  SumNumOutMax=[]  DivideOutMin=[]  DivideOutMax=[]  UdiffTsProdOutMin=[]  UdiffTsProdOutMax=[]  NTsProdOutMin=[]  NTsProdOutMax=[]  UintegralTsProdOutMin=[]  UintegralTsProdOutMax=[]  UngainTsProdOutMin=[]  UngainTsProdOutMax=[]  IntegratorContinuousStateAttributes=''  IntegratorStateMustResolveToSignalObject=off  IntegratorRTWStateStorageClass=Auto  FilterContinuousStateAttributes=''  FilterStateMustResolveToSignalObject=off  FilterRTWStateStorageClass=Auto  ParallelPVariant=InternalParameters  IdealPVariant=Disabled  IVariant=InternalParameters  DVariant=InternalParameters  IntegratorVariant=Discrete  SatVariant=Disabled  AWVariant=Passthrough  PCopyVariant=Disabled  TRVariant=Disabled  FdbkBlocksVariant=Forward  IdealPFdbkVariant=Disabled  SatFdbkVariant=Disabled  DerivativeFilterVariant=ForwardEulerFilter  NVariant=InternalParameters  NCopyVariant=Disabled  FilterICVariant=InternalICsFilter  IntegratorICVariant=InternalICs  ExternalResetVariant=Disabled  TRSumVariant=Passthrough  SumFdbkVariant=Disabled  SumVariant=Sum_PID  TsampFilterVariant=InternalTs  TsampNgainVariant=Passthrough  TsampIntegralVariant=Passthrough  ExternalSaturationOutDataTypeStr=Inherit: Same as second input  aMode=0
  Sum : Sum  Inputs=|+-
  Control Signal : Outport
  wires:
  Reference/1 -> Sum/1
  Measured Output/1 -> Sum/2
  Sum/1 -> PID/1
  PID/1 -> Control Signal/1

== system Vex-V5-Simulink-Expansion/Core Blocks/Smart Motor Controller ==
  Motor Input : Inport
  MATLAB System : MATLABSystem  System=Advanced_SmartMotorWrite  motorPort=1  scaleFactor=18:1  MotorBrakeMode=Coast  OperationMode=Advanced Control
      mask Type: Advanced_SmartMotorWrite
      mask Display:
      | color('white');
      | plot([100,100,100,100]*1,[100,100,100,100]*1);
      | plot([100,100,100,100]*0,[100,100,100,100]*0);
      | color('black');
      | image(fullfile(codertarget.vexv5.internal.getSpPkgRootDir, 'resources', 'vex-v5-motor2.png'),'center');
      | patch([0.8, 0.8, 1, 1], [0.82857, 1, 1, 0.82857], [1, 1, 1]);
      | color('blue');
      | text(99, 92, 'VEX V5 ', 'horizontalAlignment', 'right');
      | color('black');
      | text(62,12,'Port: 1','horizontalAlignment','center');
      | 
      | port_label('Input',1,'Voltage(mV)');
  wires:
  Motor Input/1 -> MATLAB System/1

== system Vex-V5-Simulink-Expansion/Core Blocks/Smart Motor Read ==
  note: Outputs
  MATLAB System1 : MATLABSystem  System=Advanced_SmartMotorRead  motorPort=1  additionalOutput=off  SampleTime=SampleTime
      mask Type: Advanced_SmartMotorRead
      mask Display:
      | color('white');
      | plot([100,100,100,100]*1,[100,100,100,100]*1);
      | plot([100,100,100,100]*0,[100,100,100,100]*0);
      | color('black');
      | image(fullfile(codertarget.vexcommon.internal.getRootDir, 'resources', 'encoder.jpg'),'center');
      | patch([0.8, 0.8, 1, 1], [0.82857, 1, 1, 0.82857], [1, 1, 1]);
      | color('blue');
      | text(75, 92, 'VEX V5 ', 'horizontalAlignment', 'right');
      | color('black');
      | text(50,15,'Port: 1','horizontalAlignment','center');
      | 
      | 
      | port_label('output',1,'Voltage');
      | port_label('output',2,'Current');
      | port_label('output',3,'Power');
      | port_label('output',4,'Torque');
      | port_label('output',5,'Efficiency');
      | port_label('output',6,'Temperature');
  Voltage : Outport
  Current : Outport  Port=2
  Power : Outport  Port=3
  Torque : Outport  Port=4
  Efficiency : Outport  Port=5
  Temperature : Outport  Port=6
  wires:
  MATLAB System1/1 -> Voltage/1
  MATLAB System1/2 -> Current/1
  MATLAB System1/3 -> Power/1
  MATLAB System1/4 -> Torque/1
  MATLAB System1/5 -> Efficiency/1
  MATLAB System1/6 -> Temperature/1
